simulink model "Nomoto2_sway"  (R2015b)
settings: Solver=ode45  StartTime=tstart  StopTime=tstop  RelTol=1e-3
values from neighbouring files (symbols this model uses):
  delta_c = deg2rad(delta_list(i))    [analyse_sway_dynamics.m]    (also in msfartoystyring.m = u(1))
  tsamp = 10    [AnalyseSpeedCharacteristis.m]    (also in AnalyseSpeedModel.m; AnalyseSurgeSpeed.m; Analyse_steadystate.m; SurgeDynamicsTest.m)
  x = lsqcurvefit(F2, x0, t, v(:,1),[],[],OPT)    [SurgeDynamicsTest.m]    (also in analyse_dynamics.m = lsqcurvefit(F3, x0, t, v(:,1),[0.09 0.2 600],[0.13 0.6 1150]; analyse_sway_dynamics.m = lsqcurvefit(F2, x0, t, v,[0 0],[],OPT))
undefined symbols (not defined in the file or in its folder): T1, T2
settings Model: ExtModeAutoUpdateStatusClock=off  Creator=christh  LastModifiedBy=Erik
settings DataIOCC: SaveFormat=Array  SignalLoggingSaveFormat=ModelDataLogs
settings OptimizationCC: ExpressionDepthLimit=2147483647  InitFltsAndDblsToZero=on
settings DebuggingCC: UnderspecifiedInitializationDetection=Classic  MergeDetectMultiDrivingBlocksExec=none  SolverPrmCheckMsg=warning  FcnCallInpInsideContextMsg=UseLocalSettings  StateNameClashWarn=warning
settings HardwareCC: ProdBitPerPointer=32  ProdLargestAtomicFloat=None  ProdIntDivRoundTo=Undefined  ProdEndianess=Unspecified  ProdWordSize=32  ProdHWDeviceType=32-bit Generic
settings GRTTargetCC: GeneratePreprocessorConditionals=Disable all  CombineOutputUpdateFcns=off  GRTInterface=on
settings ConfigComp: CovModelRefEnable=Off

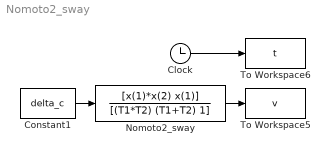
== system Nomoto2_sway ==
  Clock : Clock
  Constant1 : Constant  Value=delta_c
  Nomoto2_sway : TransferFcn  Numerator=[x(1)*x(2) x(1)]  Denominator=[(T1*T2) (T1+T2) 1]
  To Workspace5 : ToWorkspace  VariableName=v  SampleTime=tsamp
  To Workspace6 : ToWorkspace  VariableName=t  SampleTime=tsamp
  wires:
  Clock/1 -> To Workspace6/1
  Constant1/1 -> Nomoto2_sway/1
  Nomoto2_sway/1 -> To Workspace5/1
